simulink model "PMSM_FOC_DualPlant_Controller_v21"  (R2024a)
settings: Solver=FixedStepDiscrete  StartTime=0.0  StopTime=0.1  FixedStep=0.0001  RelTol=1e-3
model workspace (MAT data in the model file):
  FOC_Native_CurrentIntegratorLimit = Simulink.Parameter
  FOC_Native_CurrentIntegratorLimit.Value = 30
  FOC_Native_CurrentIntegratorLimit.Complexity = 'real'
  FOC_Native_CurrentIntegratorLimit.Dimensions = [1 1]
  FOC_Native_CurrentIntegratorLimit.DataType = 'single'
  FOC_Native_CurrentPeriod = Simulink.Parameter
  FOC_Native_CurrentPeriod.Value = 9.99999974738e-05
  FOC_Native_CurrentPeriod.Complexity = 'real'
  FOC_Native_CurrentPeriod.Dimensions = [1 1]
  FOC_Native_CurrentPeriod.DataType = 'single'
  FOC_Native_DutyMax = Simulink.Parameter
  FOC_Native_DutyMax.Value = 0.980000019073
  FOC_Native_DutyMax.Complexity = 'real'
  FOC_Native_DutyMax.Dimensions = [1 1]
  FOC_Native_DutyMax.DataType = 'single'
  FOC_Native_DutyMin = Simulink.Parameter
  FOC_Native_DutyMin.Value = 0.019999999553
  FOC_Native_DutyMin.Complexity = 'real'
  FOC_Native_DutyMin.Dimensions = [1 1]
  FOC_Native_DutyMin.DataType = 'single'
  FOC_Native_FluxPM = Simulink.Parameter
  FOC_Native_FluxPM.Value = 0.0500000007451
  FOC_Native_FluxPM.Complexity = 'real'
  FOC_Native_FluxPM.Dimensions = [1 1]
  FOC_Native_FluxPM.DataType = 'single'
  FOC_Native_IqLimit = Simulink.Parameter
  FOC_Native_IqLimit.Value = 8
  FOC_Native_IqLimit.Complexity = 'real'
  FOC_Native_IqLimit.Dimensions = [1 1]
  FOC_Native_IqLimit.DataType = 'single'
  FOC_Native_KiCurrent = Simulink.Parameter
  FOC_Native_KiCurrent.Value = 500
  FOC_Native_KiCurrent.Complexity = 'real'
  FOC_Native_KiCurrent.Dimensions = [1 1]
  FOC_Native_KiCurrent.DataType = 'single'
  FOC_Native_KiSpeed = Simulink.Parameter
  FOC_Native_KiSpeed.Value = 0.0500000007451
  FOC_Native_KiSpeed.Complexity = 'real'
  FOC_Native_KiSpeed.Dimensions = [1 1]
  FOC_Native_KiSpeed.DataType = 'single'
  FOC_Native_KpCurrent = Simulink.Parameter
  FOC_Native_KpCurrent.Value = 1
  FOC_Native_KpCurrent.Complexity = 'real'
  FOC_Native_KpCurrent.Dimensions = [1 1]
  FOC_Native_KpCurrent.DataType = 'single'
  FOC_Native_KpSpeed = Simulink.Parameter
  FOC_Native_KpSpeed.Value = 0.019999999553
  FOC_Native_KpSpeed.Complexity = 'real'
  FOC_Native_KpSpeed.Dimensions = [1 1]
  FOC_Native_KpSpeed.DataType = 'single'
  FOC_Native_Ld = Simulink.Parameter
  FOC_Native_Ld.Value = 0.0010000000475
  FOC_Native_Ld.Complexity = 'real'
  FOC_Native_Ld.Dimensions = [1 1]
  FOC_Native_Ld.DataType = 'single'
  FOC_Native_Lq = Simulink.Parameter
  FOC_Native_Lq.Value = 0.0010000000475
  FOC_Native_Lq.Complexity = 'real'
  FOC_Native_Lq.Dimensions = [1 1]
  FOC_Native_Lq.DataType = 'single'
  FOC_Native_PolePairs = Simulink.Parameter
  FOC_Native_PolePairs.Value = 4
  FOC_Native_PolePairs.Complexity = 'real'
  FOC_Native_PolePairs.Dimensions = [1 1]
  FOC_Native_PolePairs.DataType = 'single'
  FOC_Native_SpeedPeriod = Simulink.Parameter
  FOC_Native_SpeedPeriod.Value = 0.0010000000475
  FOC_Native_SpeedPeriod.Complexity = 'real'
  FOC_Native_SpeedPeriod.Dimensions = [1 1]
  FOC_Native_SpeedPeriod.DataType = 'single'
  FOC_Native_VoltageLimit = Simulink.Parameter
  FOC_Native_VoltageLimit.Value = 26
  FOC_Native_VoltageLimit.Complexity = 'real'
  FOC_Native_VoltageLimit.Dimensions = [1 1]
  FOC_Native_VoltageLimit.DataType = 'single'
  NATIVE_INV_SQRT3 = 0.577350258827
  NATIVE_RAD_S_TO_RPM = 9.54929637909
  NATIVE_RPM_TO_RAD_S = 0.104719758034
  NATIVE_SQRT3_BY2 = 0.866025388241
  PMSM_Native_B = 9.99999974738e-05
  PMSM_Native_J = 0.00200000009499
  PMSM_Native_Rs = 0.40000000596
values from neighbouring files (symbols this model uses):
  FOC_Native_CurrentIntegratorLimit = 30.0    [PMSM_FOC_Data.sldd]
  FOC_Native_CurrentPeriod = 0.0001    [PMSM_FOC_Data.sldd]
  FOC_Native_DutyMax = 0.98    [PMSM_FOC_Data.sldd]
  FOC_Native_DutyMin = 0.02    [PMSM_FOC_Data.sldd]
  FOC_Native_FluxPM = 0.05    [PMSM_FOC_Data.sldd]
  FOC_Native_IqLimit = 8.0    [PMSM_FOC_Data.sldd]
  FOC_Native_KiCurrent = 500.0    [PMSM_FOC_Data.sldd]
  FOC_Native_KiSpeed = 0.05    [PMSM_FOC_Data.sldd]
  FOC_Native_KpCurrent = 1.0    [PMSM_FOC_Data.sldd]
  FOC_Native_KpSpeed = 0.02    [PMSM_FOC_Data.sldd]
  FOC_Native_Ld = 0.001    [PMSM_FOC_Data.sldd]
  FOC_Native_Lq = 0.001    [PMSM_FOC_Data.sldd]
  FOC_Native_PolePairs = 4.0    [PMSM_FOC_Data.sldd]
  FOC_Native_SpeedPeriod = 0.001    [PMSM_FOC_Data.sldd]
  FOC_Native_VoltageLimit = 26.0    [PMSM_FOC_Data.sldd]
settings Model: Creator=18283  LastModifiedBy=18283
settings DataIOCC: SignalLogging=off
settings OptimizationCC: EnhancedBackFolding=on  PassReuseOutputArgsAs=Individual arguments  ZeroExternalMemoryAtStartup=off  ZeroInternalMemoryAtStartup=off  OptimizeBlockOrder=speed  DifferentSizesBufferReuse=on  OptimizationCustomize=off  EfficientTunableParamExpr=on
settings DebuggingCC: ParameterTunabilityLossMsg=error
settings SFSimCC: MATLABDynamicMemAlloc=off
settings RTWCC: Description=Embedded Coder  SystemTargetFile=ert.tlc  TemplateMakefile=ert_default_tmf
settings CodeAppCC: ForceParamTrailComments=on  IgnoreCustomStorageClasses=off  OperatorAnnotations=on  SimulinkDataObjDesc=on  SFDataObjDesc=on  InsertBlockDesc=on
settings ERTTargetCC: TargetLangStandard=C99 (ISO)  GenerateSampleERTMain=on  SupportNonFinite=off  ERTCustomFileTemplate=example_file_process.tlc

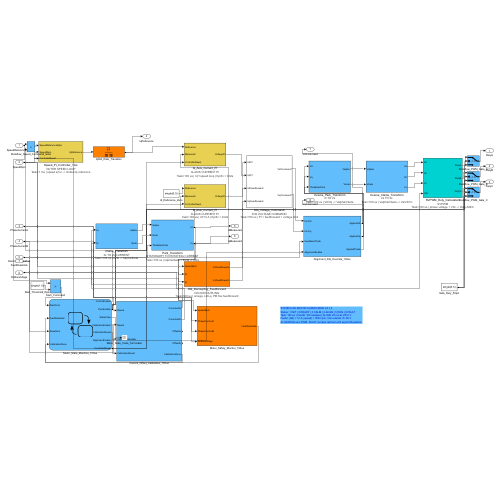
[thumbnail: Simulink's stored preview of the top-level diagram]
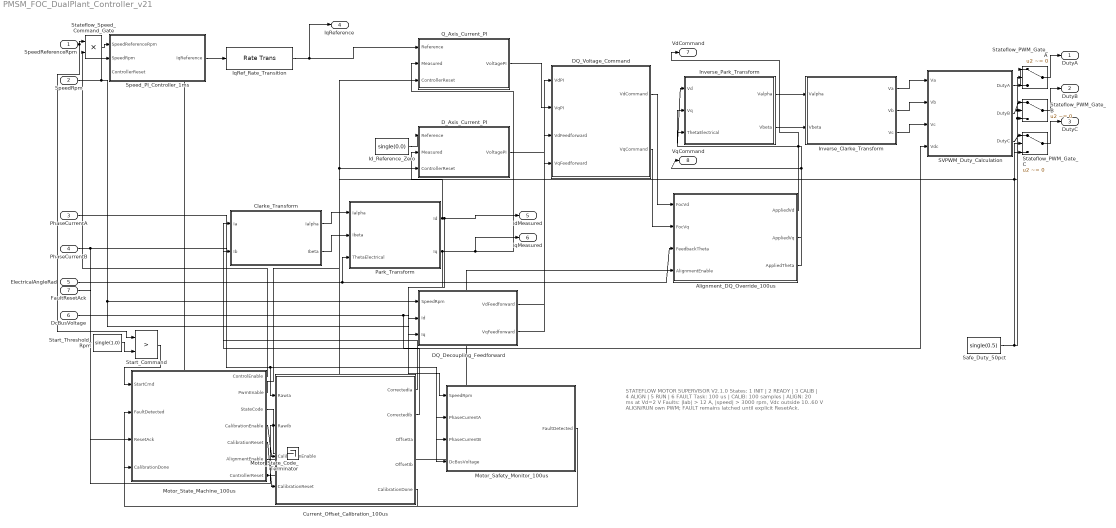
== system PMSM_FOC_DualPlant_Controller_v21 ==
  note: STATEFLOW MOTOR SUPERVISOR V2.1.0
      | States: 1 INIT | 2 READY | 3 CALIB | 4 ALIGN | 5 RUN | 6 FAULT
      | Task: 100 us | CALIB: 100 samples | ALIGN: 20 ms at Vd=2 V
      | Faults: |Iab| > 12 A, |speed| > 3000 rpm, Vdc outside 10..60 V
      | ALIGN/RUN own PWM; FAULT remains latched until explicit ResetAck.
  SpeedReferenceRpm : Inport  OutDataTypeStr=single  SampleTime=0.0001
  SpeedRpm : Inport  Port=2  OutDataTypeStr=single  SampleTime=0.0001
  PhaseCurrentA : Inport  Port=3  OutDataTypeStr=single  SampleTime=0.0001
  PhaseCurrentB : Inport  Port=4  OutDataTypeStr=single  SampleTime=0.0001
  ElectricalAngleRad : Inport  Port=5  OutDataTypeStr=single  SampleTime=0.0001
  DcBusVoltage : Inport  Port=6  OutDataTypeStr=single  SampleTime=0.0001
  FaultResetAck : Inport  Port=7  OutDataTypeStr=boolean
  Alignment_DQ_Override_100us : Subsystem
  Clarke_Transform : Subsystem  Description=|
      | 3s TO 2s CURRENT
      | Parameters: Task=100 us | Ia/Ib -> Ialpha/Ibeta
      settings: AttributesFormatString=|
      | 3s TO 2s CURRENT
      | Task=100 us | Ia/Ib -> Ialpha/Ibeta
  Current_Offset_Calibration_100us : Subsystem
  DQ_Decoupling_Feedforward : Subsystem  Description=|
      | D/Q DECOUPLING
      | Parameters: Task=100 us | omega, Ld/Lq, PM flux feedforward
      settings: AttributesFormatString=|
      | D/Q DECOUPLING
      | Task=100 us | omega, Ld/Lq, PM flux feedforward
  DQ_Voltage_Command : Subsystem  Description=|
      | D/Q VOLTAGE COMMAND
      | Parameters: Task=100 us | PI + feedforward + voltage limit
      settings: AttributesFormatString=|
      | D/Q VOLTAGE COMMAND
      | Task=100 us | PI + feedforward + voltage limit
  D_Axis_Current_PI : Subsystem  Description=|
      | D-AXIS CURRENT PI
      | Parameters: Task=100 us | Id*=0 A | Kp/Ki + limits
      settings: AttributesFormatString=|
      | D-AXIS CURRENT PI
      | Task=100 us | Id*=0 A | Kp/Ki + limits
  Id_Reference_Zero : Constant  Description=Field-oriented control d-axis current reference: Id*=0 A.  Value=single(0.0)  OutDataTypeStr=single
  Inverse_Clarke_Transform : Subsystem  Description=|
      | 2s TO 3s
      | Parameters: Task=100 us | Valpha/Vbeta -> Va/Vb/Vc
      settings: AttributesFormatString=|
      | 2s TO 3s
      | Task=100 us | Valpha/Vbeta -> Va/Vb/Vc
  Inverse_Park_Transform : Subsystem  Description=|
      | 2r TO 2s
      | Parameters: Task=100 us | Vd/Vq -> Valpha/Vbeta
      settings: AttributesFormatString=|
      | 2r TO 2s
      | Task=100 us | Vd/Vq -> Valpha/Vbeta
  IqRef_Rate_Transition : RateTransition  Description=Explicit deterministic transfer from 1 ms speed task to 100 us current task.  OutPortSampleTime=0.0001
  Motor_Safety_Monitor_100us : Subsystem
  Motor_State_Code_Terminator : Terminator
  Motor_State_Machine_100us : Stateflow chart  TreatAsAtomicUnit=on
  Park_Transform : Subsystem  Description=|
      | STATIONARY TO ROTATING CURRENT
      | Parameters: Task=100 us | Ialpha/Ibeta + theta -> Id/Iq
      settings: AttributesFormatString=|
      | STATIONARY TO ROTATING CURRENT
      | Task=100 us | Ialpha/Ibeta + theta -> Id/Iq
  Q_Axis_Current_PI : Subsystem  Description=|
      | Q-AXIS CURRENT PI
      | Parameters: Task=100 us | Iq*=speed loop | Kp/Ki + limits
      settings: AttributesFormatString=|
      | Q-AXIS CURRENT PI
      | Task=100 us | Iq*=speed loop | Kp/Ki + limits
  SVPWM_Duty_Calculation : Subsystem  Description=|
      | SVPWM
      | Parameters: Task=100 us | phase voltage + Vdc -> Duty A/B/C
      settings: AttributesFormatString=|
      | SVPWM
      | Task=100 us | phase voltage + Vdc -> Duty A/B/C
  Safe_Duty_50pct : Constant  Value=single(0.5)  OutDataTypeStr=single
  Speed_PI_Controller_1ms : Subsystem  Description=|
      | OUTER SPEED LOOP
      | Parameters: Task=1 ms | speed error -> limited Iq reference
      settings: AttributesFormatString=|
      | OUTER SPEED LOOP
      | Task=1 ms | speed error -> limited Iq reference
  Start_Command : RelationalOperator  Operator=>  OutDataTypeStr=boolean  RndMeth=Simplest  InputSameDT=off
  Start_Threshold_Rpm : Constant  Value=single(1.0)  OutDataTypeStr=single
  Stateflow_PWM_Gate_A : Switch  Criteria=u2 ~= 0  SaturateOnIntegerOverflow=off  InputSameDT=off
  Stateflow_PWM_Gate_B : Switch  Criteria=u2 ~= 0  SaturateOnIntegerOverflow=off  InputSameDT=off
  Stateflow_PWM_Gate_C : Switch  Criteria=u2 ~= 0  SaturateOnIntegerOverflow=off  InputSameDT=off
  Stateflow_Speed_Command_Gate : Product  Inputs=**
  DutyA : Outport  OutDataTypeStr=single
  DutyB : Outport  Port=2  OutDataTypeStr=single
  DutyC : Outport  Port=3  OutDataTypeStr=single
  IqReference : Outport  Port=4  OutDataTypeStr=single
  IdMeasured : Outport  Port=5  OutDataTypeStr=single
  IqMeasured : Outport  Port=6  OutDataTypeStr=single
  VdCommand : Outport  Port=7  OutDataTypeStr=single
  VqCommand : Outport  Port=8  OutDataTypeStr=single
  wires:
  SpeedRpm/1 -> DQ_Decoupling_Feedforward/1(SpeedRpm), Motor_Safety_Monitor_100us/1(SpeedRpm), Speed_PI_Controller_1ms/2(SpeedRpm)
  Speed_PI_Controller_1ms/1(IqReference) -> IqRef_Rate_Transition/1
  IqRef_Rate_Transition/1 -> Q_Axis_Current_PI/1(Reference), IqReference/1
  Clarke_Transform/1(Ialpha) -> Park_Transform/1(Ialpha)
  Clarke_Transform/2(Ibeta) -> Park_Transform/2(Ibeta)
  ElectricalAngleRad/1 -> Park_Transform/3(ThetaElectrical), Alignment_DQ_Override_100us/3(FeedbackTheta)
  Id_Reference_Zero/1 -> D_Axis_Current_PI/1(Reference)
  Park_Transform/1(Id) -> IdMeasured/1, DQ_Decoupling_Feedforward/2(Id), D_Axis_Current_PI/2(Measured)
  Park_Transform/2(Iq) -> Q_Axis_Current_PI/2(Measured), IqMeasured/1, DQ_Decoupling_Feedforward/3(Iq)
  D_Axis_Current_PI/1(VoltagePI) -> DQ_Voltage_Command/1(VdPI)
  Q_Axis_Current_PI/1(VoltagePI) -> DQ_Voltage_Command/2(VqPI)
  DQ_Decoupling_Feedforward/1(VdFeedforward) -> DQ_Voltage_Command/3(VdFeedforward)
  DQ_Decoupling_Feedforward/2(VqFeedforward) -> DQ_Voltage_Command/4(VqFeedforward)
  Inverse_Park_Transform/1(Valpha) -> Inverse_Clarke_Transform/1(Valpha)
  Inverse_Park_Transform/2(Vbeta) -> Inverse_Clarke_Transform/2(Vbeta)
  Inverse_Clarke_Transform/1(Va) -> SVPWM_Duty_Calculation/1(Va)
  Inverse_Clarke_Transform/2(Vb) -> SVPWM_Duty_Calculation/2(Vb)
  Inverse_Clarke_Transform/3(Vc) -> SVPWM_Duty_Calculation/3(Vc)
  DcBusVoltage/1 -> SVPWM_Duty_Calculation/4(Vdc), Motor_Safety_Monitor_100us/4(DcBusVoltage)
  SpeedReferenceRpm/1 -> Start_Command/1, Stateflow_Speed_Command_Gate/1
  Start_Threshold_Rpm/1 -> Start_Command/2
  Start_Command/1 -> Motor_State_Machine_100us/1(StartCmd)
  PhaseCurrentA/1 -> Motor_Safety_Monitor_100us/2(PhaseCurrentA), Current_Offset_Calibration_100us/1(RawIa)
  PhaseCurrentB/1 -> Motor_Safety_Monitor_100us/3(PhaseCurrentB), Current_Offset_Calibration_100us/2(RawIb)
  Motor_Safety_Monitor_100us/1(FaultDetected) -> Motor_State_Machine_100us/2(FaultDetected)
  FaultResetAck/1 -> Motor_State_Machine_100us/3(ResetAck)
  Motor_State_Machine_100us/4(CalibrationEnable) -> Current_Offset_Calibration_100us/3(CalibrationEnable)
  Motor_State_Machine_100us/5(CalibrationReset) -> Current_Offset_Calibration_100us/4(CalibrationReset)
  Current_Offset_Calibration_100us/5(CalibrationDone) -> Motor_State_Machine_100us/4(CalibrationDone)
  Current_Offset_Calibration_100us/1(CorrectedIa) -> Clarke_Transform/1(Ia)
  Current_Offset_Calibration_100us/2(CorrectedIb) -> Clarke_Transform/2(Ib)
  Motor_State_Machine_100us/1(ControlEnable) -> Stateflow_Speed_Command_Gate/2
  Stateflow_Speed_Command_Gate/1 -> Speed_PI_Controller_1ms/1(SpeedReferenceRpm)
  Motor_State_Machine_100us/7(ControllerReset) -> D_Axis_Current_PI/3(ControllerReset), Q_Axis_Current_PI/3(ControllerReset), Speed_PI_Controller_1ms/3(ControllerReset)
  DQ_Voltage_Command/1(VdCommand) -> Alignment_DQ_Override_100us/1(FocVd)
  DQ_Voltage_Command/2(VqCommand) -> Alignment_DQ_Override_100us/2(FocVq)
  Motor_State_Machine_100us/6(AlignmentEnable) -> Alignment_DQ_Override_100us/4(AlignmentEnable)
  Alignment_DQ_Override_100us/1(AppliedVd) -> Inverse_Park_Transform/1(Vd), VdCommand/1
  Alignment_DQ_Override_100us/2(AppliedVq) -> Inverse_Park_Transform/2(Vq), VqCommand/1
  Alignment_DQ_Override_100us/3(AppliedTheta) -> Inverse_Park_Transform/3(ThetaElectrical)
  SVPWM_Duty_Calculation/1(DutyA) -> Stateflow_PWM_Gate_A/1
  Motor_State_Machine_100us/2(PwmEnable) -> Stateflow_PWM_Gate_A/2, Stateflow_PWM_Gate_B/2, Stateflow_PWM_Gate_C/2
  Safe_Duty_50pct/1 -> Stateflow_PWM_Gate_A/3, Stateflow_PWM_Gate_B/3, Stateflow_PWM_Gate_C/3
  SVPWM_Duty_Calculation/2(DutyB) -> Stateflow_PWM_Gate_B/1
  SVPWM_Duty_Calculation/3(DutyC) -> Stateflow_PWM_Gate_C/1
  Stateflow_PWM_Gate_A/1 -> DutyA/1
  Stateflow_PWM_Gate_B/1 -> DutyB/1
  Stateflow_PWM_Gate_C/1 -> DutyC/1
  Motor_State_Machine_100us/3(StateCode) -> Motor_State_Code_Terminator/1

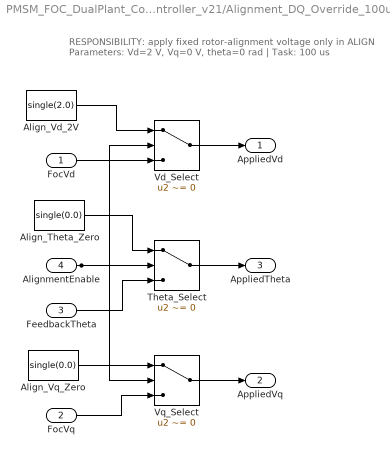
== system PMSM_FOC_DualPlant_Controller_v21/Alignment_DQ_Override_100us ==
  note: RESPONSIBILITY: apply fixed rotor-alignment voltage only in ALIGN
      | Parameters: Vd=2 V, Vq=0 V, theta=0 rad | Task: 100 us
  FocVd : Inport
  FocVq : Inport  Port=2
  FeedbackTheta : Inport  Port=3
  AlignmentEnable : Inport  Port=4
  Align_Theta_Zero : Constant  Value=single(0.0)  OutDataTypeStr=single
  Align_Vd_2V : Constant  Value=single(2.0)  OutDataTypeStr=single
  Align_Vq_Zero : Constant  Value=single(0.0)  OutDataTypeStr=single
  Theta_Select : Switch  Criteria=u2 ~= 0  SaturateOnIntegerOverflow=off  InputSameDT=off
  Vd_Select : Switch  Criteria=u2 ~= 0  SaturateOnIntegerOverflow=off  InputSameDT=off
  Vq_Select : Switch  Criteria=u2 ~= 0  SaturateOnIntegerOverflow=off  InputSameDT=off
  AppliedVd : Outport
  AppliedVq : Outport  Port=2
  AppliedTheta : Outport  Port=3
  wires:
  FeedbackTheta/1 -> Theta_Select/3
  Align_Vd_2V/1 -> Vd_Select/1
  FocVd/1 -> Vd_Select/3
  Align_Theta_Zero/1 -> Theta_Select/1
  Vd_Select/1 -> AppliedVd/1
  AlignmentEnable/1 -> Vd_Select/2, Vq_Select/2, Theta_Select/2
  Align_Vq_Zero/1 -> Vq_Select/1
  FocVq/1 -> Vq_Select/3
  Theta_Select/1 -> AppliedTheta/1
  Vq_Select/1 -> AppliedVq/1

== system PMSM_FOC_DualPlant_Controller_v21/Clarke_Transform ==
  note: RESPONSIBILITY: two-current Clarke transform
      | Ialpha = Ia; Ibeta = (Ia + 2*Ib)/sqrt(3)
      | Parameter: NATIVE_INV_SQRT3
  Ia : Inport  OutDataTypeStr=single
  Ib : Inport  Port=2  OutDataTypeStr=single
  Ia_Plus_2Ib : Sum
  Ib_x2 : Gain  Gain=single(2.0)
  InvSqrt3 : Gain  Gain=NATIVE_INV_SQRT3
  Ialpha : Outport  OutDataTypeStr=single
  Ibeta : Outport  Port=2  OutDataTypeStr=single
  wires:
  Ia/1 -> Ialpha/1, Ia_Plus_2Ib/1
  Ib/1 -> Ib_x2/1
  Ib_x2/1 -> Ia_Plus_2Ib/2
  Ia_Plus_2Ib/1 -> InvSqrt3/1
  InvSqrt3/1 -> Ibeta/1

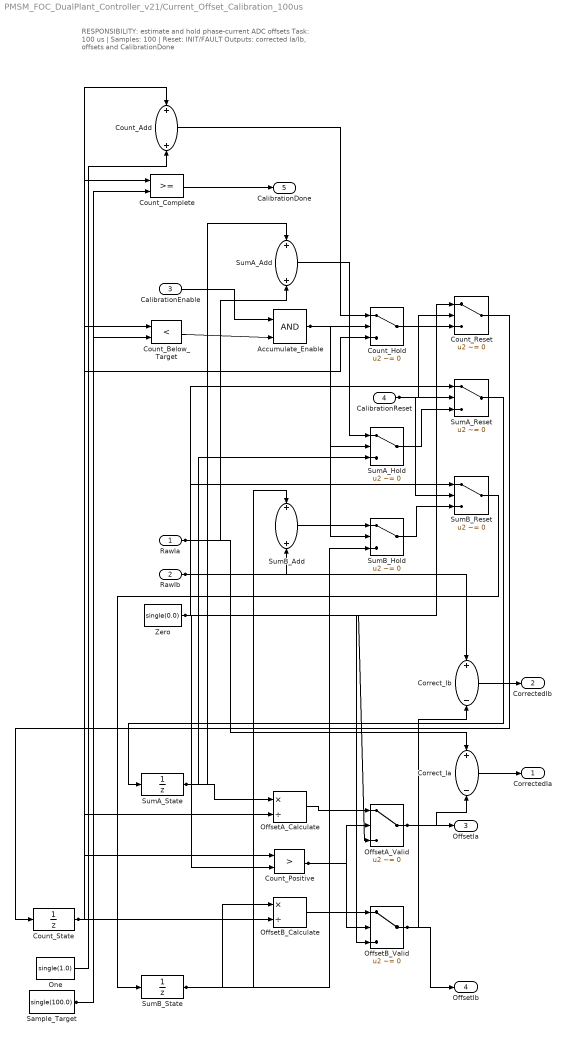
== system PMSM_FOC_DualPlant_Controller_v21/Current_Offset_Calibration_100us ==
  note: RESPONSIBILITY: estimate and hold phase-current ADC offsets
      | Task: 100 us | Samples: 100 | Reset: INIT/FAULT
      | Outputs: corrected Ia/Ib, offsets and CalibrationDone
  RawIa : Inport
  RawIb : Inport  Port=2
  CalibrationEnable : Inport  Port=3
  CalibrationReset : Inport  Port=4
  Accumulate_Enable : Logic  AllPortsSameDT=off  OutDataTypeStr=boolean
  Correct_Ia : Sum  Inputs=+-
  Correct_Ib : Sum  Inputs=+-
  Count_Add : Sum
  Count_Below_Target : RelationalOperator  Operator=<  OutDataTypeStr=boolean  RndMeth=Simplest  InputSameDT=off
  Count_Complete : RelationalOperator  OutDataTypeStr=boolean  RndMeth=Simplest  InputSameDT=off
  Count_Hold : Switch  Criteria=u2 ~= 0  SaturateOnIntegerOverflow=off  InputSameDT=off
  Count_Positive : RelationalOperator  Operator=>  OutDataTypeStr=boolean  RndMeth=Simplest  InputSameDT=off
  Count_Reset : Switch  Criteria=u2 ~= 0  SaturateOnIntegerOverflow=off  InputSameDT=off
  Count_State : UnitDelay  InitialCondition=single(0.0)  SampleTime=0.0001  HasFrameUpgradeWarning=on
  OffsetA_Calculate : Product  Inputs=*/
  OffsetA_Valid : Switch  Criteria=u2 ~= 0  SaturateOnIntegerOverflow=off  InputSameDT=off
  OffsetB_Calculate : Product  Inputs=*/
  OffsetB_Valid : Switch  Criteria=u2 ~= 0  SaturateOnIntegerOverflow=off  InputSameDT=off
  One : Constant  Value=single(1.0)  OutDataTypeStr=single
  Sample_Target : Constant  Value=single(100.0)  OutDataTypeStr=single
  SumA_Add : Sum
  SumA_Hold : Switch  Criteria=u2 ~= 0  SaturateOnIntegerOverflow=off  InputSameDT=off
  SumA_Reset : Switch  Criteria=u2 ~= 0  SaturateOnIntegerOverflow=off  InputSameDT=off
  SumA_State : UnitDelay  InitialCondition=single(0.0)  SampleTime=0.0001  HasFrameUpgradeWarning=on
  SumB_Add : Sum
  SumB_Hold : Switch  Criteria=u2 ~= 0  SaturateOnIntegerOverflow=off  InputSameDT=off
  SumB_Reset : Switch  Criteria=u2 ~= 0  SaturateOnIntegerOverflow=off  InputSameDT=off
  SumB_State : UnitDelay  InitialCondition=single(0.0)  SampleTime=0.0001  HasFrameUpgradeWarning=on
  Zero : Constant  Value=single(0.0)  OutDataTypeStr=single
  CorrectedIa : Outport
  CorrectedIb : Outport  Port=2
  OffsetIa : Outport  Port=3
  OffsetIb : Outport  Port=4
  CalibrationDone : Outport  Port=5
  wires:
  CalibrationEnable/1 -> Accumulate_Enable/1
  OffsetB_Calculate/1 -> OffsetB_Valid/1
  Count_Complete/1 -> CalibrationDone/1
  Count_State/1 -> Count_Hold/3, OffsetA_Calculate/2, OffsetB_Calculate/2, Count_Complete/1, Count_Positive/1, Count_Below_Target/1, Count_Add/1
  Count_Below_Target/1 -> Accumulate_Enable/2
  Count_Add/1 -> Count_Hold/1
  One/1 -> Count_Add/2
  Sample_Target/1 -> Count_Below_Target/2, Count_Complete/2
  RawIa/1 -> SumA_Add/2, Correct_Ia/1
  RawIb/1 -> SumB_Add/2, Correct_Ib/1
  Count_Reset/1 -> Count_State/1
  Zero/1 -> SumA_Reset/1, SumB_Reset/1, OffsetA_Valid/3, OffsetB_Valid/3, Count_Positive/2, Count_Reset/1
  SumA_State/1 -> SumA_Hold/3, SumA_Add/1, OffsetA_Calculate/1
  CalibrationReset/1 -> SumA_Reset/2, SumB_Reset/2, Count_Reset/2
  SumB_State/1 -> SumB_Add/1, SumB_Hold/3, OffsetB_Calculate/1
  SumA_Add/1 -> SumA_Hold/1
  Accumulate_Enable/1 -> SumB_Hold/2, Count_Hold/2, SumA_Hold/2
  SumA_Hold/1 -> SumA_Reset/3
  SumB_Add/1 -> SumB_Hold/1
  OffsetA_Calculate/1 -> OffsetA_Valid/1
  Count_Positive/1 -> OffsetA_Valid/2, OffsetB_Valid/2
  Count_Hold/1 -> Count_Reset/3
  SumB_Hold/1 -> SumB_Reset/3
  OffsetA_Valid/1 -> Correct_Ia/2, OffsetIa/1
  OffsetB_Valid/1 -> Correct_Ib/2, OffsetIb/1
  SumA_Reset/1 -> SumA_State/1
  SumB_Reset/1 -> SumB_State/1
  Correct_Ib/1 -> CorrectedIb/1
  Correct_Ia/1 -> CorrectedIa/1

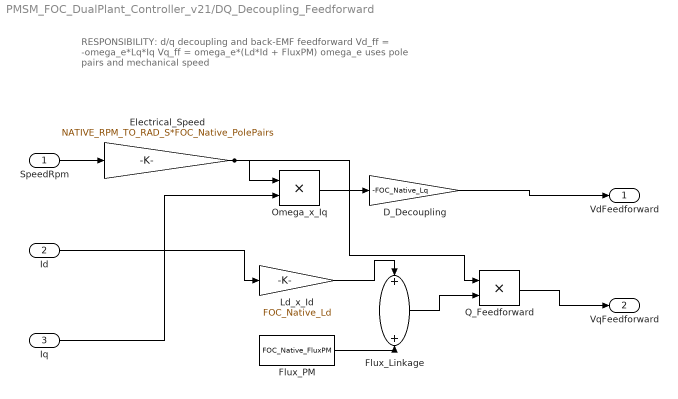
== system PMSM_FOC_DualPlant_Controller_v21/DQ_Decoupling_Feedforward ==
  note: RESPONSIBILITY: d/q decoupling and back-EMF feedforward
      | Vd_ff = -omega_e*Lq*Iq
      | Vq_ff = omega_e*(Ld*Id + FluxPM)
      | omega_e uses pole pairs and mechanical speed
  SpeedRpm : Inport  OutDataTypeStr=single
  Id : Inport  Port=2  OutDataTypeStr=single
  Iq : Inport  Port=3  OutDataTypeStr=single
  D_Decoupling : Gain  Gain=-FOC_Native_Lq
  Electrical_Speed : Gain  Gain=NATIVE_RPM_TO_RAD_S*FOC_Native_PolePairs
  Flux_Linkage : Sum
  Flux_PM : Constant  Value=FOC_Native_FluxPM  OutDataTypeStr=single
  Ld_x_Id : Gain  Gain=FOC_Native_Ld
  Omega_x_Iq : Product  Inputs=**
  Q_Feedforward : Product  Inputs=**
  VdFeedforward : Outport  OutDataTypeStr=single
  VqFeedforward : Outport  Port=2  OutDataTypeStr=single
  wires:
  SpeedRpm/1 -> Electrical_Speed/1
  Electrical_Speed/1 -> Omega_x_Iq/1, Q_Feedforward/1
  Iq/1 -> Omega_x_Iq/2
  Omega_x_Iq/1 -> D_Decoupling/1
  D_Decoupling/1 -> VdFeedforward/1
  Id/1 -> Ld_x_Id/1
  Ld_x_Id/1 -> Flux_Linkage/1
  Flux_PM/1 -> Flux_Linkage/2
  Flux_Linkage/1 -> Q_Feedforward/2
  Q_Feedforward/1 -> VqFeedforward/1

== system PMSM_FOC_DualPlant_Controller_v21/DQ_Voltage_Command ==
  note: RESPONSIBILITY: synthesize bounded d/q voltage commands
      | Vd = sat(Vd_PI + Vd_ff); Vq = sat(Vq_PI + Vq_ff)
      | Limit: +/-FOC_Native_VoltageLimit
  VdPI : Inport  OutDataTypeStr=single
  VqPI : Inport  Port=2  OutDataTypeStr=single
  VdFeedforward : Inport  Port=3  OutDataTypeStr=single
  VqFeedforward : Inport  Port=4  OutDataTypeStr=single
  Vd_Limit : Saturate  UpperLimit=FOC_Native_VoltageLimit  LowerLimit=-FOC_Native_VoltageLimit
  Vd_Raw : Sum
  Vq_Limit : Saturate  UpperLimit=FOC_Native_VoltageLimit  LowerLimit=-FOC_Native_VoltageLimit
  Vq_Raw : Sum
  VdCommand : Outport  OutDataTypeStr=single
  VqCommand : Outport  Port=2  OutDataTypeStr=single
  wires:
  VdPI/1 -> Vd_Raw/1
  VdFeedforward/1 -> Vd_Raw/2
  VqPI/1 -> Vq_Raw/1
  VqFeedforward/1 -> Vq_Raw/2
  Vd_Raw/1 -> Vd_Limit/1
  Vq_Raw/1 -> Vq_Limit/1
  Vd_Limit/1 -> VdCommand/1
  Vq_Limit/1 -> VqCommand/1

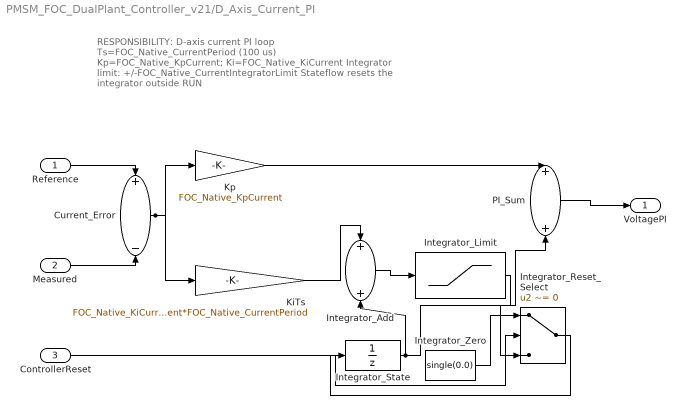
== system PMSM_FOC_DualPlant_Controller_v21/D_Axis_Current_PI ==
  note: RESPONSIBILITY: D-axis current PI loop
      | Ts=FOC_Native_CurrentPeriod (100 us)
      | Kp=FOC_Native_KpCurrent; Ki=FOC_Native_KiCurrent
      | Integrator limit: +/-FOC_Native_CurrentIntegratorLimit
      | Stateflow resets the integrator outside RUN
  Reference : Inport  OutDataTypeStr=single
  Measured : Inport  Port=2  OutDataTypeStr=single
  ControllerReset : Inport  Port=3  OutDataTypeStr=boolean
  Current_Error : Sum  Inputs=+-
  Integrator_Add : Sum
  Integrator_Limit : Saturate  UpperLimit=FOC_Native_CurrentIntegratorLimit  LowerLimit=-FOC_Native_CurrentIntegratorLimit
  Integrator_Reset_Select : Switch  Criteria=u2 ~= 0  SaturateOnIntegerOverflow=off  InputSameDT=off
  Integrator_State : UnitDelay  InitialCondition=single(0.0)  SampleTime=0.0001  HasFrameUpgradeWarning=on
  Integrator_Zero : Constant  Value=single(0.0)  OutDataTypeStr=single
  KiTs : Gain  Gain=FOC_Native_KiCurrent*FOC_Native_CurrentPeriod
  Kp : Gain  Gain=FOC_Native_KpCurrent
  PI_Sum : Sum
  VoltagePI : Outport  OutDataTypeStr=single
  wires:
  Reference/1 -> Current_Error/1
  Measured/1 -> Current_Error/2
  Current_Error/1 -> Kp/1, KiTs/1
  KiTs/1 -> Integrator_Add/1
  Integrator_State/1 -> Integrator_Add/2, PI_Sum/2
  Integrator_Add/1 -> Integrator_Limit/1
  Integrator_Zero/1 -> Integrator_Reset_Select/1
  ControllerReset/1 -> Integrator_Reset_Select/2
  Integrator_Limit/1 -> Integrator_Reset_Select/3
  Integrator_Reset_Select/1 -> Integrator_State/1
  Kp/1 -> PI_Sum/1
  PI_Sum/1 -> VoltagePI/1

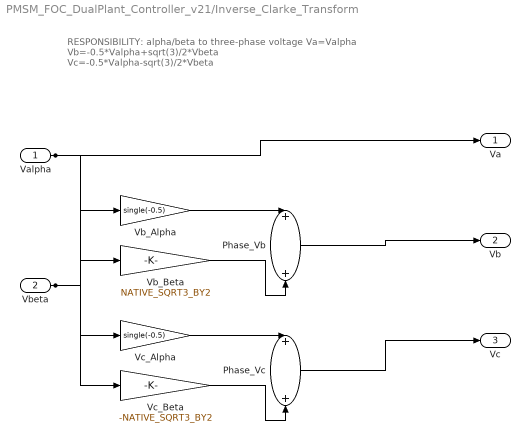
== system PMSM_FOC_DualPlant_Controller_v21/Inverse_Clarke_Transform ==
  note: RESPONSIBILITY: alpha/beta to three-phase voltage
      | Va=Valpha
      | Vb=-0.5*Valpha+sqrt(3)/2*Vbeta
      | Vc=-0.5*Valpha-sqrt(3)/2*Vbeta
  Valpha : Inport  OutDataTypeStr=single
  Vbeta : Inport  Port=2  OutDataTypeStr=single
  Phase_Vb : Sum
  Phase_Vc : Sum
  Vb_Alpha : Gain  Gain=single(-0.5)
  Vb_Beta : Gain  Gain=NATIVE_SQRT3_BY2
  Vc_Alpha : Gain  Gain=single(-0.5)
  Vc_Beta : Gain  Gain=-NATIVE_SQRT3_BY2
  Va : Outport  OutDataTypeStr=single
  Vb : Outport  Port=2  OutDataTypeStr=single
  Vc : Outport  Port=3  OutDataTypeStr=single
  wires:
  Valpha/1 -> Va/1, Vb_Alpha/1, Vc_Alpha/1
  Vbeta/1 -> Vb_Beta/1, Vc_Beta/1
  Vb_Alpha/1 -> Phase_Vb/1
  Vb_Beta/1 -> Phase_Vb/2
  Phase_Vb/1 -> Vb/1
  Vc_Alpha/1 -> Phase_Vc/1
  Vc_Beta/1 -> Phase_Vc/2
  Phase_Vc/1 -> Vc/1

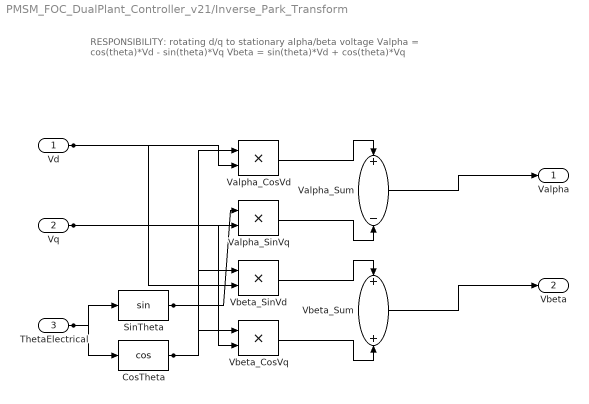
== system PMSM_FOC_DualPlant_Controller_v21/Inverse_Park_Transform ==
  note: RESPONSIBILITY: rotating d/q to stationary alpha/beta voltage
      | Valpha = cos(theta)*Vd - sin(theta)*Vq
      | Vbeta = sin(theta)*Vd + cos(theta)*Vq
  Vd : Inport  OutDataTypeStr=single
  Vq : Inport  Port=2  OutDataTypeStr=single
  ThetaElectrical : Inport  Port=3  OutDataTypeStr=single
  CosTheta : Trigonometry  Operator=cos
  SinTheta : Trigonometry
  Valpha_CosVd : Product  Inputs=**
  Valpha_SinVq : Product  Inputs=**
  Valpha_Sum : Sum  Inputs=+-
  Vbeta_CosVq : Product  Inputs=**
  Vbeta_SinVd : Product  Inputs=**
  Vbeta_Sum : Sum
  Valpha : Outport  OutDataTypeStr=single
  Vbeta : Outport  Port=2  OutDataTypeStr=single
  wires:
  ThetaElectrical/1 -> SinTheta/1, CosTheta/1
  CosTheta/1 -> Valpha_CosVd/1, Vbeta_CosVq/1
  Vd/1 -> Valpha_CosVd/2, Vbeta_SinVd/2
  SinTheta/1 -> Valpha_SinVq/1, Vbeta_SinVd/1
  Vq/1 -> Valpha_SinVq/2, Vbeta_CosVq/2
  Valpha_CosVd/1 -> Valpha_Sum/1
  Valpha_SinVq/1 -> Valpha_Sum/2
  Valpha_Sum/1 -> Valpha/1
  Vbeta_SinVd/1 -> Vbeta_Sum/1
  Vbeta_CosVq/1 -> Vbeta_Sum/2
  Vbeta_Sum/1 -> Vbeta/1

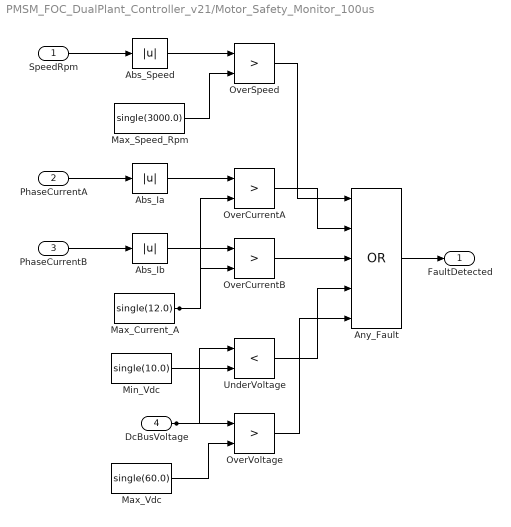
== system PMSM_FOC_DualPlant_Controller_v21/Motor_Safety_Monitor_100us ==
  SpeedRpm : Inport
  PhaseCurrentA : Inport  Port=2
  PhaseCurrentB : Inport  Port=3
  DcBusVoltage : Inport  Port=4
  Abs_Ia : Abs  SaturateOnIntegerOverflow=off
  Abs_Ib : Abs  SaturateOnIntegerOverflow=off
  Abs_Speed : Abs  SaturateOnIntegerOverflow=off
  Any_Fault : Logic  Operator=OR  Inputs=5  AllPortsSameDT=off  OutDataTypeStr=boolean
  Max_Current_A : Constant  Value=single(12.0)  OutDataTypeStr=single
  Max_Speed_Rpm : Constant  Value=single(3000.0)  OutDataTypeStr=single
  Max_Vdc : Constant  Value=single(60.0)  OutDataTypeStr=single
  Min_Vdc : Constant  Value=single(10.0)  OutDataTypeStr=single
  OverCurrentA : RelationalOperator  Operator=>  OutDataTypeStr=boolean  RndMeth=Simplest  InputSameDT=off
  OverCurrentB : RelationalOperator  Operator=>  OutDataTypeStr=boolean  RndMeth=Simplest  InputSameDT=off
  OverSpeed : RelationalOperator  Operator=>  OutDataTypeStr=boolean  RndMeth=Simplest  InputSameDT=off
  OverVoltage : RelationalOperator  Operator=>  OutDataTypeStr=boolean  RndMeth=Simplest  InputSameDT=off
  UnderVoltage : RelationalOperator  Operator=<  OutDataTypeStr=boolean  RndMeth=Simplest  InputSameDT=off
  FaultDetected : Outport
  wires:
  Max_Speed_Rpm/1 -> OverSpeed/2
  SpeedRpm/1 -> Abs_Speed/1
  OverVoltage/1 -> Any_Fault/5
  PhaseCurrentA/1 -> Abs_Ia/1
  Abs_Ib/1 -> OverCurrentB/1
  PhaseCurrentB/1 -> Abs_Ib/1
  Abs_Speed/1 -> OverSpeed/1
  Abs_Ia/1 -> OverCurrentA/1
  Max_Current_A/1 -> OverCurrentA/2, OverCurrentB/2
  Min_Vdc/1 -> UnderVoltage/2
  DcBusVoltage/1 -> OverVoltage/1, UnderVoltage/1
  Max_Vdc/1 -> OverVoltage/2
  OverSpeed/1 -> Any_Fault/1
  OverCurrentA/1 -> Any_Fault/2
  OverCurrentB/1 -> Any_Fault/3
  UnderVoltage/1 -> Any_Fault/4
  Any_Fault/1 -> FaultDetected/1

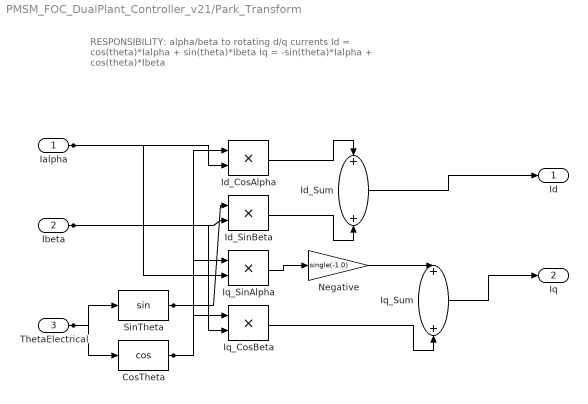
== system PMSM_FOC_DualPlant_Controller_v21/Park_Transform ==
  note: RESPONSIBILITY: alpha/beta to rotating d/q currents
      | Id = cos(theta)*Ialpha + sin(theta)*Ibeta
      | Iq = -sin(theta)*Ialpha + cos(theta)*Ibeta
  Ialpha : Inport  OutDataTypeStr=single
  Ibeta : Inport  Port=2  OutDataTypeStr=single
  ThetaElectrical : Inport  Port=3  OutDataTypeStr=single
  CosTheta : Trigonometry  Operator=cos
  Id_CosAlpha : Product  Inputs=**
  Id_SinBeta : Product  Inputs=**
  Id_Sum : Sum
  Iq_CosBeta : Product  Inputs=**
  Iq_SinAlpha : Product  Inputs=**
  Iq_Sum : Sum
  Negative : Gain  Gain=single(-1.0)
  SinTheta : Trigonometry
  Id : Outport  OutDataTypeStr=single
  Iq : Outport  Port=2  OutDataTypeStr=single
  wires:
  ThetaElectrical/1 -> SinTheta/1, CosTheta/1
  CosTheta/1 -> Id_CosAlpha/1, Iq_CosBeta/1
  Ialpha/1 -> Id_CosAlpha/2, Iq_SinAlpha/2
  SinTheta/1 -> Id_SinBeta/1, Iq_SinAlpha/1
  Ibeta/1 -> Id_SinBeta/2, Iq_CosBeta/2
  Id_CosAlpha/1 -> Id_Sum/1
  Id_SinBeta/1 -> Id_Sum/2
  Id_Sum/1 -> Id/1
  Iq_SinAlpha/1 -> Negative/1
  Negative/1 -> Iq_Sum/1
  Iq_CosBeta/1 -> Iq_Sum/2
  Iq_Sum/1 -> Iq/1

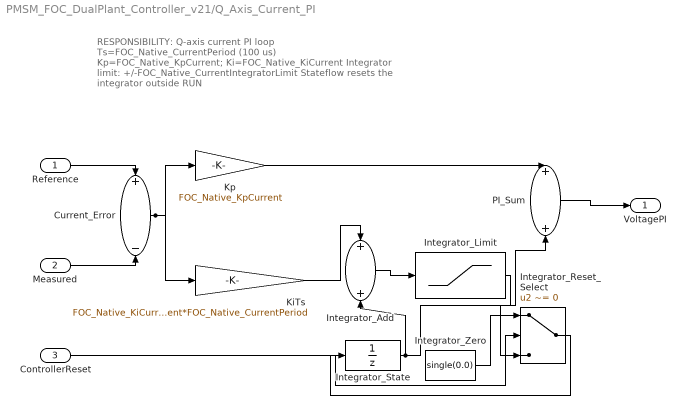
== system PMSM_FOC_DualPlant_Controller_v21/Q_Axis_Current_PI ==
  note: RESPONSIBILITY: Q-axis current PI loop
      | Ts=FOC_Native_CurrentPeriod (100 us)
      | Kp=FOC_Native_KpCurrent; Ki=FOC_Native_KiCurrent
      | Integrator limit: +/-FOC_Native_CurrentIntegratorLimit
      | Stateflow resets the integrator outside RUN
  Reference : Inport  OutDataTypeStr=single
  Measured : Inport  Port=2  OutDataTypeStr=single
  ControllerReset : Inport  Port=3  OutDataTypeStr=boolean
  Current_Error : Sum  Inputs=+-
  Integrator_Add : Sum
  Integrator_Limit : Saturate  UpperLimit=FOC_Native_CurrentIntegratorLimit  LowerLimit=-FOC_Native_CurrentIntegratorLimit
  Integrator_Reset_Select : Switch  Criteria=u2 ~= 0  SaturateOnIntegerOverflow=off  InputSameDT=off
  Integrator_State : UnitDelay  InitialCondition=single(0.0)  SampleTime=0.0001  HasFrameUpgradeWarning=on
  Integrator_Zero : Constant  Value=single(0.0)  OutDataTypeStr=single
  KiTs : Gain  Gain=FOC_Native_KiCurrent*FOC_Native_CurrentPeriod
  Kp : Gain  Gain=FOC_Native_KpCurrent
  PI_Sum : Sum
  VoltagePI : Outport  OutDataTypeStr=single
  wires:
  Reference/1 -> Current_Error/1
  Measured/1 -> Current_Error/2
  Current_Error/1 -> Kp/1, KiTs/1
  KiTs/1 -> Integrator_Add/1
  Integrator_State/1 -> Integrator_Add/2, PI_Sum/2
  Integrator_Add/1 -> Integrator_Limit/1
  Integrator_Zero/1 -> Integrator_Reset_Select/1
  ControllerReset/1 -> Integrator_Reset_Select/2
  Integrator_Limit/1 -> Integrator_Reset_Select/3
  Integrator_Reset_Select/1 -> Integrator_State/1
  Kp/1 -> PI_Sum/1
  PI_Sum/1 -> VoltagePI/1

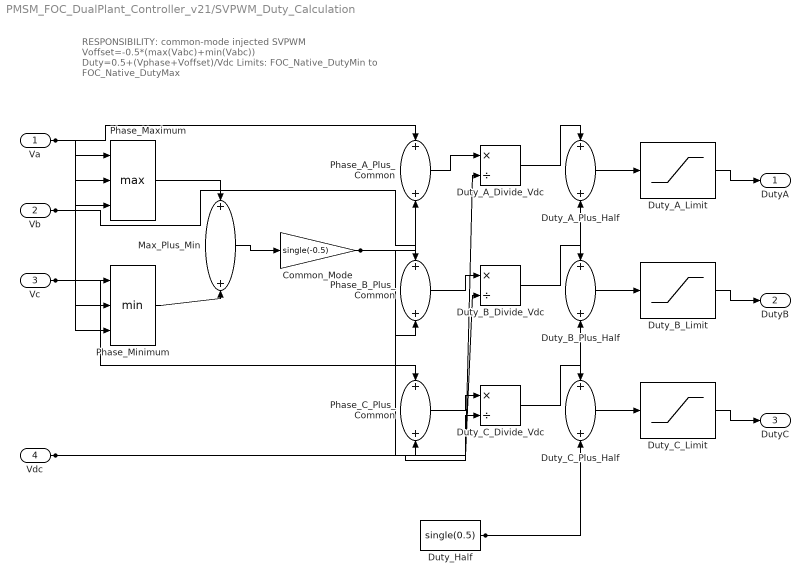
== system PMSM_FOC_DualPlant_Controller_v21/SVPWM_Duty_Calculation ==
  note: RESPONSIBILITY: common-mode injected SVPWM
      | Voffset=-0.5*(max(Vabc)+min(Vabc))
      | Duty=0.5+(Vphase+Voffset)/Vdc
      | Limits: FOC_Native_DutyMin to FOC_Native_DutyMax
  Va : Inport  OutDataTypeStr=single
  Vb : Inport  Port=2  OutDataTypeStr=single
  Vc : Inport  Port=3  OutDataTypeStr=single
  Vdc : Inport  Port=4  OutDataTypeStr=single
  Common_Mode : Gain  Gain=single(-0.5)
  Duty_A_Divide_Vdc : Product  Inputs=*/
  Duty_A_Limit : Saturate  UpperLimit=FOC_Native_DutyMax  LowerLimit=FOC_Native_DutyMin
  Duty_A_Plus_Half : Sum
  Duty_B_Divide_Vdc : Product  Inputs=*/
  Duty_B_Limit : Saturate  UpperLimit=FOC_Native_DutyMax  LowerLimit=FOC_Native_DutyMin
  Duty_B_Plus_Half : Sum
  Duty_C_Divide_Vdc : Product  Inputs=*/
  Duty_C_Limit : Saturate  UpperLimit=FOC_Native_DutyMax  LowerLimit=FOC_Native_DutyMin
  Duty_C_Plus_Half : Sum
  Duty_Half : Constant  Value=single(0.5)  OutDataTypeStr=single
  Max_Plus_Min : Sum
  Phase_A_Plus_Common : Sum
  Phase_B_Plus_Common : Sum
  Phase_C_Plus_Common : Sum
  Phase_Maximum : MinMax  Function=max  Inputs=3
  Phase_Minimum : MinMax  Inputs=3
  DutyA : Outport  OutDataTypeStr=single
  DutyB : Outport  Port=2  OutDataTypeStr=single
  DutyC : Outport  Port=3  OutDataTypeStr=single
  wires:
  Va/1 -> Phase_A_Plus_Common/1, Phase_Maximum/1, Phase_Minimum/1
  Common_Mode/1 -> Phase_A_Plus_Common/2, Phase_B_Plus_Common/2, Phase_C_Plus_Common/2
  Phase_A_Plus_Common/1 -> Duty_A_Divide_Vdc/1
  Vdc/1 -> Duty_A_Divide_Vdc/2, Duty_B_Divide_Vdc/2, Duty_C_Divide_Vdc/2
  Duty_A_Divide_Vdc/1 -> Duty_A_Plus_Half/1
  Duty_Half/1 -> Duty_A_Plus_Half/2, Duty_B_Plus_Half/2, Duty_C_Plus_Half/2
  Duty_A_Plus_Half/1 -> Duty_A_Limit/1
  Duty_A_Limit/1 -> DutyA/1
  Vb/1 -> Phase_B_Plus_Common/1, Phase_Maximum/2, Phase_Minimum/2
  Phase_B_Plus_Common/1 -> Duty_B_Divide_Vdc/1
  Duty_B_Divide_Vdc/1 -> Duty_B_Plus_Half/1
  Duty_B_Plus_Half/1 -> Duty_B_Limit/1
  Duty_B_Limit/1 -> DutyB/1
  Vc/1 -> Phase_C_Plus_Common/1, Phase_Maximum/3, Phase_Minimum/3
  Phase_C_Plus_Common/1 -> Duty_C_Divide_Vdc/1
  Duty_C_Divide_Vdc/1 -> Duty_C_Plus_Half/1
  Duty_C_Plus_Half/1 -> Duty_C_Limit/1
  Duty_C_Limit/1 -> DutyC/1
  Phase_Maximum/1 -> Max_Plus_Min/1
  Phase_Minimum/1 -> Max_Plus_Min/2
  Max_Plus_Min/1 -> Common_Mode/1

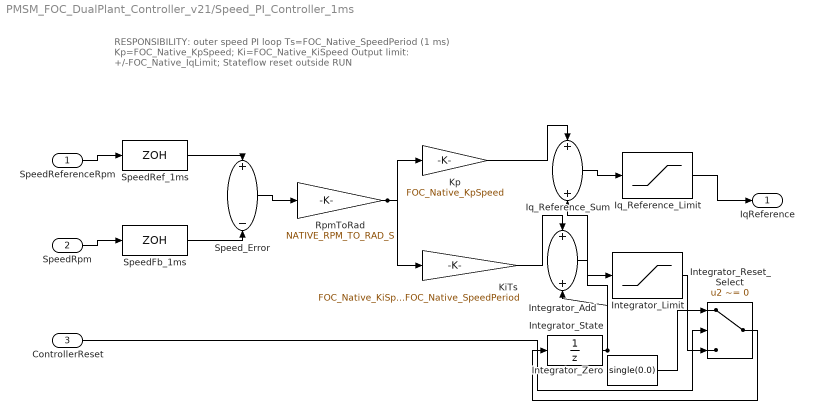
== system PMSM_FOC_DualPlant_Controller_v21/Speed_PI_Controller_1ms ==
  note: RESPONSIBILITY: outer speed PI loop
      | Ts=FOC_Native_SpeedPeriod (1 ms)
      | Kp=FOC_Native_KpSpeed; Ki=FOC_Native_KiSpeed
      | Output limit: +/-FOC_Native_IqLimit; Stateflow reset outside RUN
  SpeedReferenceRpm : Inport  OutDataTypeStr=single
  SpeedRpm : Inport  Port=2  OutDataTypeStr=single
  ControllerReset : Inport  Port=3  OutDataTypeStr=boolean
  Integrator_Add : Sum
  Integrator_Limit : Saturate  UpperLimit=FOC_Native_IqLimit  LowerLimit=-FOC_Native_IqLimit
  Integrator_Reset_Select : Switch  Criteria=u2 ~= 0  SaturateOnIntegerOverflow=off  InputSameDT=off
  Integrator_State : UnitDelay  InitialCondition=single(0.0)  SampleTime=0.001  HasFrameUpgradeWarning=on
  Integrator_Zero : Constant  Value=single(0.0)  OutDataTypeStr=single
  Iq_Reference_Limit : Saturate  UpperLimit=FOC_Native_IqLimit  LowerLimit=-FOC_Native_IqLimit
  Iq_Reference_Sum : Sum
  KiTs : Gain  Gain=FOC_Native_KiSpeed*FOC_Native_SpeedPeriod
  Kp : Gain  Gain=FOC_Native_KpSpeed
  RpmToRad : Gain  Gain=NATIVE_RPM_TO_RAD_S
  SpeedFb_1ms : ZeroOrderHold  SampleTime=0.001
  SpeedRef_1ms : ZeroOrderHold  SampleTime=0.001
  Speed_Error : Sum  Inputs=+-
  IqReference : Outport  OutDataTypeStr=single
  wires:
  SpeedReferenceRpm/1 -> SpeedRef_1ms/1
  SpeedRpm/1 -> SpeedFb_1ms/1
  SpeedRef_1ms/1 -> Speed_Error/1
  SpeedFb_1ms/1 -> Speed_Error/2
  Speed_Error/1 -> RpmToRad/1
  RpmToRad/1 -> Kp/1, KiTs/1
  KiTs/1 -> Integrator_Add/1
  Integrator_State/1 -> Integrator_Add/2, Iq_Reference_Sum/2
  Integrator_Add/1 -> Integrator_Limit/1
  Integrator_Zero/1 -> Integrator_Reset_Select/1
  ControllerReset/1 -> Integrator_Reset_Select/2
  Integrator_Limit/1 -> Integrator_Reset_Select/3
  Integrator_Reset_Select/1 -> Integrator_State/1
  Kp/1 -> Iq_Reference_Sum/1
  Iq_Reference_Sum/1 -> Iq_Reference_Limit/1
  Iq_Reference_Limit/1 -> IqReference/1

== stateflow chart PMSM_FOC_DualPlant_Controller_v21/Motor_State_Machine_100us ==
  settings: updateMethod=DISCRETE  sampleTime=0.0001
  state SUPERVISED
    state INIT
      entry:
      ControlEnable = 0;
      PwmEnable = 0;
      StateCode = 1;
      CalibrationEnable = 0;
      CalibrationReset = 1;
      AlignmentEnable = 0;
      ControllerReset = 1;
    state READY
      entry:
      ControlEnable = 0;
      PwmEnable = 0;
      StateCode = 2;
      CalibrationEnable = 0;
      CalibrationReset = 0;
      AlignmentEnable = 0;
      ControllerReset = 1;
    state CALIB
      entry:
      ControlEnable = 0;
      PwmEnable = 0;
      StateCode = 3;
      CalibrationEnable = 1;
      CalibrationReset = 0;
      AlignmentEnable = 0;
      ControllerReset = 1;
    state ALIGN
      entry:
      ControlEnable = 0;
      PwmEnable = 1;
      StateCode = 4;
      CalibrationEnable = 0;
      CalibrationReset = 0;
      AlignmentEnable = 1;
      ControllerReset = 1;
    state RUN
      entry:
      ControlEnable = 1;
      PwmEnable = 1;
      StateCode = 5;
      CalibrationEnable = 0;
      CalibrationReset = 0;
      AlignmentEnable = 0;
      ControllerReset = 0;
    INIT -> READY : after(1,tick)
    READY -> CALIB : [StartCmd]
    CALIB -> ALIGN [order 1] : [CalibrationDone]
    ALIGN -> RUN [order 1] : after(200,tick)
    ALIGN -> INIT [order 2] : [!StartCmd]
    RUN -> INIT : [!StartCmd]
  state FAULT
    entry:
    ControlEnable = 0;
    PwmEnable = 0;
    StateCode = 6;
    CalibrationEnable = 0;
    CalibrationReset = 1;
    AlignmentEnable = 0;
    ControllerReset = 1;
  (default) -> INIT
  CALIB -> FAULT [order 2] : after(150,tick)
  SUPERVISED -> FAULT : [FaultDetected]
  FAULT -> INIT : [ResetAck && !FaultDetected && !StartCmd]
  data: StartCmd input boolean; FaultDetected input boolean; ResetAck input boolean; CalibrationDone input boolean; ControlEnable output boolean; PwmEnable output boolean; StateCode output uint8; CalibrationEnable output boolean; CalibrationReset output boolean; AlignmentEnable output boolean; ControllerReset output boolean
